simulink model "DC_motor"  (R2021b)
settings: Solver=ode3  StartTime=0.0  StopTime=10.0  FixedStep=1e-4  RelTol=1e-3
values from neighbouring files (symbols this model uses):
  J_motor = 0.000610871894223    [var_10.mat]
  L_phase = 0.00332259990587    [var_10.mat]
  psi = 0.0961787034043    [var_10.mat]
  R_phase = 0.753894801324    [var_10.mat]
  U_nom = 48    [var_10.mat]
settings Model: Creator=Denis  LastModifiedBy=Denis

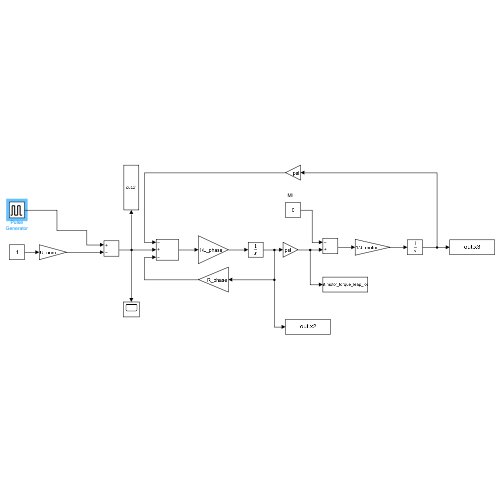
[thumbnail: Simulink's stored preview of the top-level diagram]
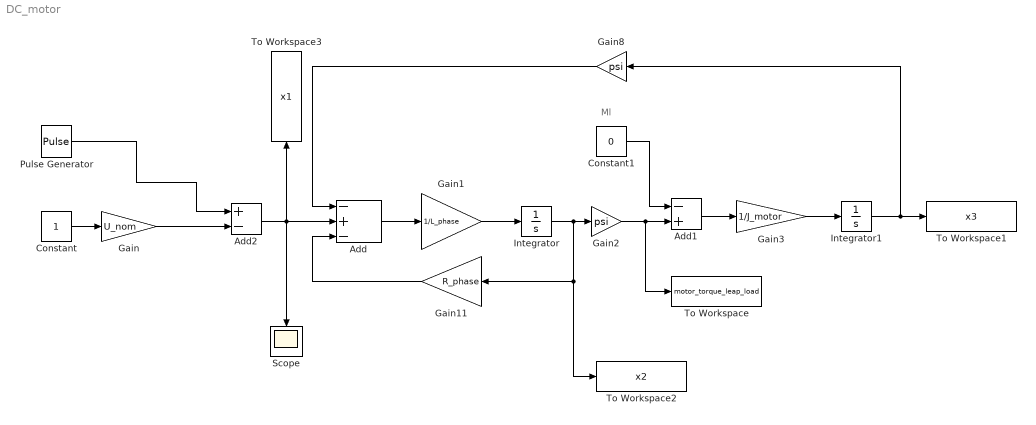
== system DC_motor ==
  note: Ml
  Add : Sum  Inputs=-+-
  Add1 : Sum  Inputs=-+
  Add2 : Sum  Inputs=+-
  Constant : Constant
  Constant1 : Constant  Value=0
  Gain : Gain  Gain=U_nom
  Gain1 : Gain  Gain=1/L_phase
  Gain11 : Gain  Gain=R_phase
  Gain2 : Gain  Gain=psi
  Gain3 : Gain  Gain=1/J_motor
  Gain8 : Gain  Gain=psi
  Integrator : Integrator
  Integrator1 : Integrator
  Pulse Generator : DiscretePulseGenerator  PulseType=Time based  Amplitude=2*U_nom  PulseWidth=50
  Scope : Scope
  To Workspace : ToWorkspace  VariableName=motor_torque_leap_load  SaveFormat=Timeseries  SampleTime=-1
  To Workspace1 : ToWorkspace  VariableName=x3  SaveFormat=Timeseries  SampleTime=-1
  To Workspace2 : ToWorkspace  VariableName=x2  SaveFormat=Timeseries  SampleTime=-1
  To Workspace3 : ToWorkspace  VariableName=x1  SaveFormat=Timeseries  SampleTime=-1
  wires:
  Gain11/1 -> Add/3
  Gain8/1 -> Add/1
  Gain2/1 -> To Workspace/1, Add1/2
  Add1/1 -> Gain3/1
  Constant/1 -> Gain/1
  Constant1/1 -> Add1/1
  Gain3/1 -> Integrator1/1
  Integrator1/1 -> Gain8/1, To Workspace1/1
  Integrator/1 -> To Workspace2/1, Gain11/1, Gain2/1
  Gain1/1 -> Integrator/1
  Add/1 -> Gain1/1
  Pulse Generator/1 -> Add2/1
  Add2/1 -> Add/2, Scope/1, To Workspace3/1
  Gain/1 -> Add2/2
